simulink model "SensorNoise"  (R2017b)
settings: Solver=ode1  StartTime=0.0  StopTime=40  FixedStep=0.002  RelTol=1e-3  EnableMultiTasking=on
PreLoadFcn:
  | quanser_aero_lqr
libraries: quanser_aero x1, quarc_library x1
settings Model: SimulationMode=external  ExtModeTrigDuration=15000  Creator=MLevis  LastModifiedBy=craigr1
settings SolverCC: PositivePriorityOrder=on
settings DataIOCC: SaveFormat=Array
settings OptimizationCC: LifeSpan=inf
settings DebuggingCC: SolverPrmCheckMsg=warning  SFUnexpectedBacktrackingDiag=warning  SFNoUnconditionalDefaultTransitionDiag=warning  SFExecutionAtInitializationDiag=none
settings HardwareCC: ProdBitPerPointer=32  ProdBitPerSizeT=32  ProdBitPerPtrDiffT=32  ProdLargestAtomicFloat=None  ProdIntDivRoundTo=Undefined  ProdEndianess=Unspecified  ProdWordSize=32  ProdHWDeviceType=32-bit Generic
settings ModelReferenceCC: PropagateSignalLabelsOutOfModel=off
settings RTWCC: SystemTargetFile=quarc_win64.tlc  TemplateMakefile=quarc_default_tmf  Description=QUARC Win64 Target
settings CodeAppCC: StateflowObjectComments=on
settings STFCustomTargetCC: TargetPreCompLibLocation=C:\PROGRA~3\QUARC\lib\2017b\win64\release  ConcurrentExecutionCompliant=on  GeneratePreprocessorConditionals=Disable all  SystemTargetFile=quarc_win64.tlc
settings GRTTargetCC: TargetPreCompLibLocation=C:\PROGRA~3\QUARC\lib\2017b\win64\release  TargetLangStandard=C89/C90 (ANSI)  ParMdlRefBuildCompliant=off  CompOptLevelCompliant=off  GeneratePreprocessorConditionals=Disable all  CombineOutputUpdateFcns=off  MatFileLogging=off  CPPClassGenCompliant=off  GRTInterface=on  UseToolchainInfoCompliant=off  ExtMode=on  ExtModeMexFile=quarc_comm
settings ConfigComp: CovMetricSettings=dw  CovHtmlReporting=on  CovSaveCumulativeToWorkspaceVar=on  CovSaveSingleToWorkspaceVar=on  CovExternalEMLEnable=off  CovSFcnEnable=off

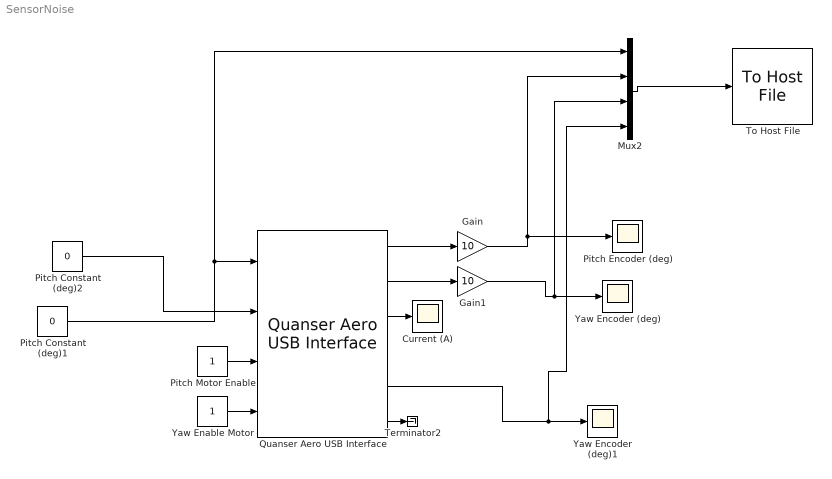
== system SensorNoise ==
  Current (A) : Scope
  Gain : Gain  Gain=10
  Gain1 : Gain  Gain=10
  Mux2 : Mux
  Pitch Constant (deg)1 : Constant  Value=0
  Pitch Constant (deg)2 : Constant  Value=0
  Pitch Encoder (deg) : Scope
  Pitch Motor Enable : Constant
  Quanser Aero USB Interface : quanser_aero/Quanser Aero USB Interface
  Terminator2 : Terminator
  To Host File : quarc_library/Sinks/To Host/To Host File  file_name=SensorNoise_NoInput2.mat  variable_name=Data  decimation=1  sample_time=-1  file_format=MAT-file v.4  options=No header or footer  append=off  final_file_name=SensorNoise_NoInput2.mat  bitrate=2000000
  Yaw Enable Motor : Constant
  Yaw Encoder (deg) : Scope
  Yaw Encoder (deg)1 : Scope
  wires:
  Pitch Motor Enable/1 -> Quanser Aero USB Interface/3
  Yaw Enable Motor/1 -> Quanser Aero USB Interface/4
  Quanser Aero USB Interface/3 -> Current (A)/1
  Quanser Aero USB Interface/5 -> Mux2/4, Yaw Encoder (deg)1/1
  Quanser Aero USB Interface/6 -> Terminator2/1
  Mux2/1 -> To Host File/1
  Pitch Constant (deg)1/1 -> Mux2/1, Quanser Aero USB Interface/1
  Quanser Aero USB Interface/1 -> Gain/1
  Gain/1 -> Mux2/2, Pitch Encoder (deg)/1
  Quanser Aero USB Interface/2 -> Gain1/1
  Gain1/1 -> Yaw Encoder (deg)/1, Mux2/3
  Pitch Constant (deg)2/1 -> Quanser Aero USB Interface/2
